simulink model "regenerative_damper_with_battery"  (R2017a)
settings: Solver=ode45  StartTime=0.0  StopTime=0.05  MaxStep=1e-5  RelTol=1e-4
libraries: powerlib_meascontrol x17, fl_lib x12, nesl_utility x11, pe_lib x4, elec_lib x1, powerlib x1
settings Model: Creator=k1506456  LastModifiedBy=k1506456

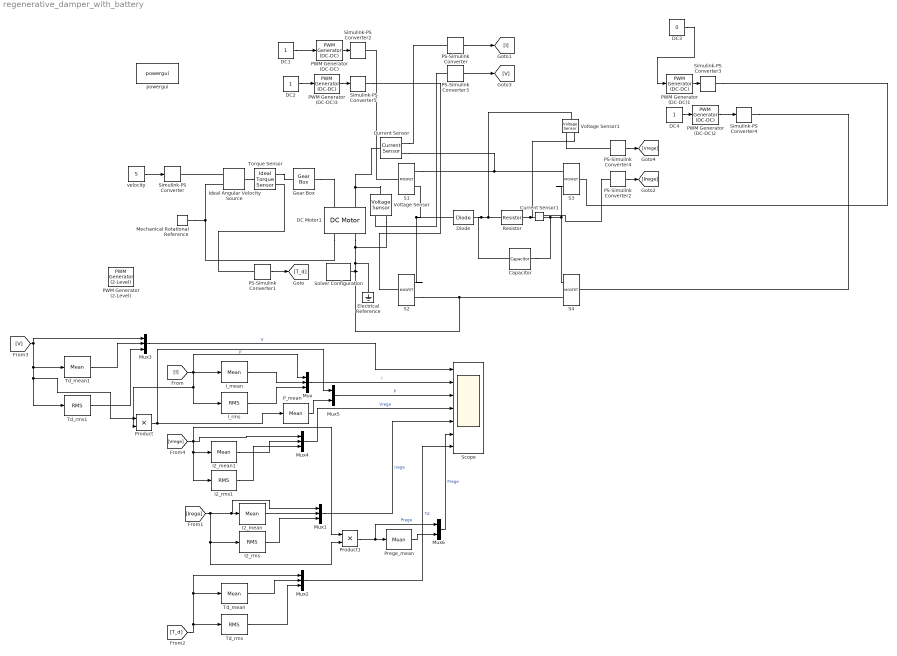
== system regenerative_damper_with_battery ==
  Capacitor : fl_lib/Electrical/Electrical Elements/Capacitor  c=220 uF  r=1e-6 Ohm  g=0 1/Ohm  i_specify=off  i_priority=None  i=0 A  i_nominal_specify=off  i_nominal_unit=A  i_nominal_value=1  v_specify=off  v_priority=None  v=0 V  v_nominal_specify=off  v_nominal_unit=V  v_nominal_value=1  vc_specify=off  vc_priority=High  vc=0 V  vc_nominal_specify=off  vc_nominal_unit=V  vc_nominal_value=1
  Current Sensor : fl_lib/Electrical/Electrical Sensors/Current Sensor
  Current Sensor1 : fl_lib/Electrical/Electrical Sensors/Current Sensor
  DC Motor1 : elec_lib/Actuators & Drivers/Rotational Actuators/DC Motor  parameterization=1  Ra=21.2 Ohm  La=1.37 mH  emf_or_torque=1  Kv=0.00222222 V/rpm  Ki=0.0212 N*m/A  T_stall=2.4e-4 N*m  w_max=1.91e+4 rpm  w_rated=1.5e+4 rpm  P_rated=0.08 W  V_rated=1.5 V  J=4.2 g*cm^2  lam_param=2  lam=0 N*m/(rad/s)  i_noload=8.81 mA  V_i_noload=24 V  speed0=100 rad/s  alpha=0.00393 1/K  Tmeas=25 degC  thermal_mass=100 J/K  initial_temperature=25 degC
  DC1 : Constant
  DC2 : Constant
  DC3 : Constant  Value=0
  DC4 : Constant
  Diode : fl_lib/Electrical/Electrical Elements/Diode  Vf=0.1 V  Ron=0.001 Ohm  Goff=1e-8 1/Ohm  i_specify=off  i_priority=None  i=0 A  i_nominal_specify=off  i_nominal_unit=A  i_nominal_value=1  v_specify=off  v_priority=None  v=0 V  v_nominal_specify=off  v_nominal_unit=V  v_nominal_value=1
  Electrical Reference : fl_lib/Electrical/Electrical Elements/Electrical Reference
  Gear Box : fl_lib/Mechanical/Mechanisms/Gear Box  ratio=1/20  t_in_specify=off  t_in_priority=None  t_in=0 N*m  t_in_nominal_specify=off  t_in_nominal_unit=N*m  t_in_nominal_value=1  t_out_specify=off  t_out_priority=None  t_out=0 N*m  t_out_nominal_specify=off  t_out_nominal_unit=N*m  t_out_nominal_value=1
  I2_mean : powerlib_meascontrol/Measurements/Mean  Freq=100  Vinit=0  Ts=0
  I2_mean1 : powerlib_meascontrol/Measurements/Mean  Freq=50  Vinit=0  Ts=0
  I2_rms : powerlib_meascontrol/Measurements/RMS  TrueRMS=on  Freq=50  RMSInit=0  Ts=0
  I2_rms1 : powerlib_meascontrol/Measurements/RMS  TrueRMS=on  Freq=50  RMSInit=0  Ts=0
  I_mean : powerlib_meascontrol/Measurements/Mean  Freq=50  Vinit=0  Ts=0
  I_rms : powerlib_meascontrol/Measurements/RMS  TrueRMS=on  Freq=50  RMSInit=0  Ts=0
  Ideal Angular Velocity Source : fl_lib/Mechanical/Mechanical Sources/Ideal Angular Velocity Source
  Mechanical Rotational Reference : fl_lib/Mechanical/Rotational Elements/Mechanical Rotational Reference
  Mux{,1..4} (5 alike) : Mux  Inputs=3
  Mux5 : Mux  Inputs=2
  Mux6 : Mux  Inputs=2
  PS-Simulink Converter{,1..4} (5 alike) : nesl_utility/PS-Simulink Converter  PhysicalDomain=network_engine_domain  SubClassName=ps_output  LeftPortType=input  RightPortType=output  PseudoPeriodic=off  Frequencies=[]  Unit=1  AffineConversion=off
  PWM Generator (2-Level) : powerlib_meascontrol/Pulse & Signal Generators/PWM Generator (2-Level)  ModulatorType=Three-phase bridge (6 pulses)  ModulatorMode=Unsynchronized  Fc=5000  Pc=90  nF=27  MinMax="[ -1  1 ]"  SamplingTechnique=Natural  ModulatingSignals=off  m=0.8  Freq=60  Phase=0  Ts=0  ShowCarrierOutport=off
      settings: SourceProductName=Simscape Power Systems
  PWM Generator (DC-DC) : powerlib_meascontrol/Pulse & Signal Generators/PWM Generator (DC-DC)  Fsw=1000  Ts=0
  PWM Generator (DC-DC)1 : powerlib_meascontrol/Pulse & Signal Generators/PWM Generator (DC-DC)  Fsw=1000  Ts=0
  PWM Generator (DC-DC)2 : powerlib_meascontrol/Pulse & Signal Generators/PWM Generator (DC-DC)  Fsw=1000  Ts=0
  PWM Generator (DC-DC)3 : powerlib_meascontrol/Pulse & Signal Generators/PWM Generator (DC-DC)  Fsw=5000  Ts=0
  P_mean : powerlib_meascontrol/Measurements/Mean  Freq=50  Vinit=0  Ts=0
  Prege_mean : powerlib_meascontrol/Measurements/Mean  Freq=50  Vinit=0  Ts=0
  Product : Product
  Product1 : Product
  Resistor : fl_lib/Electrical/Electrical Elements/Resistor  R=21.2 Ohm  i_specify=off  i_priority=None  i=0 A  i_nominal_specify=off  i_nominal_unit=A  i_nominal_value=1  v_specify=off  v_priority=None  v=0 V  v_nominal_specify=off  v_nominal_unit=V  v_nominal_value=1
  S{1..4} (4 alike) : pe_lib/Semiconductors/Fundamental Components/MOSFET  Rds=0.001 Ohm  Goff=1e-6 1/Ohm  Vth=0.8 V  diode_param=2  diode_Vf=0.8 V  diode_Ron=0.001 Ohm  diode_Goff=1e-5 1/Ohm  diode_C=5e-8 F  diode_iRM=-235 A  diode_iF=300 A  diode_idot=-50 A/us  diode_trr_param=1  diode_trr_factor=3  diode_trr=15 us  diode_Qrr=1.5e+3 s*uA  thermal_loss_option=2  Voff=300 V  Tau=1e-4 s  Tj=[ 298.15 398.15 ] K  Iout_scalar=600 A  Eon_scalar=0.02286 J  Eoff_scalar=0.01714 J  Von_scalar=2.7 V  Iout_data=[ 0 10 50 100 200 400 600 ] A  Eon_data=[ 0 2.9e-4 0.00143 0.00286 0.00571 0.01314 0.02286; 0 5.7e-4 0.00263 0.00514 0.01029 0.02057 0.03029 ] J  Eoff_data=[ 0 2.1e-4 0.00107 0.00214 0.00429 0.009859999999999999 0.01714; 0 4.3e-4 0.00197 0.00386 0.00771 0.01543 0.02271 ] J  Von_data=[ 0 1.1 1.3 1.45 1.75 2.25 2.7; 0 1 1.15 1.35 1.7 2.35 3 ] V
      settings: SourceProductName=Simscape Power Systems  SourceProductBaseCode=PS
  Scope : Scope  NumInputPorts=7
  Simulink-PS Converter : nesl_utility/Simulink-PS Converter  PhysicalDomain=network_engine_domain  SubClassName=ps_input  LeftPortType=input  RightPortType=output  PseudoPeriodic=off  Frequencies=[]  NoiseDistribution=none  NoiseParameters=[]  Unit=rad/s  AffineConversion=off  FilteringAndDerivatives=provide  SimscapeFilterOrder=1  InputFilterTimeConstant=0.001  UdotUserProvided=0
  Simulink-PS Converter{2..5} (4 alike) : nesl_utility/Simulink-PS Converter  PhysicalDomain=network_engine_domain  SubClassName=ps_input  LeftPortType=input  RightPortType=output  PseudoPeriodic=off  Frequencies=[]  NoiseDistribution=none  NoiseParameters=[]  Unit=V  AffineConversion=off  FilteringAndDerivatives=provide  SimscapeFilterOrder=1  InputFilterTimeConstant=0.001  UdotUserProvided=0
  Solver Configuration : nesl_utility/Solver Configuration  PhysicalDomain=network_engine_domain  SubClassName=solver  LeftPortType=input  RightPortType=generic  Accelerate=off  Tones=[]  Harmonics=[]  SimulateNoise=off  Profile=off  UseLocalSampling=off  EnableSwitchedLinearOptims=on  FrequencyDomain=off  UseCCode=off  RelTol=0.001  AbsTol=1e-06  MinStep=1e-09  ToWorkspace=off  RevertToSquareIcSolve=off  NumHomotopyIterations=100  PhasorMode=off  PhasorModeNumHarmonics=1  OverrideAbsTol=off  DoDC=off  ResidualTolerance=1e-09  UseLocalSolver=off  LocalSolverChoice=NE_BACKWARD_EULER_ADVANCER  LocalSolverSampleTime=0.001  DoFixedCost=off  MaxNonlinIter=3  MaxModeIter=2  LinearAlgebra=Sparse  DelaysMemoryBudget=1024  AutomaticFiltering=on  FilteringTimeConstant=0.001
  Td_mean : powerlib_meascontrol/Measurements/Mean  Freq=100  Vinit=0  Ts=0
  Td_mean1 : powerlib_meascontrol/Measurements/Mean  Freq=50  Vinit=0  Ts=0
  Td_rms : powerlib_meascontrol/Measurements/RMS  TrueRMS=on  Freq=50  RMSInit=0  Ts=0
  Td_rms1 : powerlib_meascontrol/Measurements/RMS  TrueRMS=on  Freq=50  RMSInit=0  Ts=0
  Torque Sensor : fl_lib/Mechanical/Mechanical Sensors/Ideal Torque Sensor
  Voltage Sensor : fl_lib/Electrical/Electrical Sensors/Voltage Sensor
  Voltage Sensor1 : fl_lib/Electrical/Electrical Sensors/Voltage Sensor
  powergui : powerlib/powergui  Priority=1  SimulationMode=Continuous  SampleTime=5e-6  frequency=60  Iterations=50  frequencyindice=0  Pbase=100e6  ErrMax=1e-4  UnitsV=kV  UnitsW=MW  buscounter=0  FunctionMessages=off  echomessages=off  EnableUseOfTLC=off  CurrentSourceSwitches=off  DisableSnubberDevices=off  DisableRonSwitches=off  DisableVfSwitches=off  DisplayEquations=off  SolverType=Tustin/Backward Euler (TBE)  Interpol=off  ExternalGateDelay=off  methode=off  Ts=100  x0status=blocks  SPID=on  SwTol=0  HookPort=off  RestoreLinks=warning  ResistiveCurrentMeasurement=off  Frange=[0:2:500]  Ylog=off  Xlog=on  ShowGrid=off  save=off  variable=ZData  structure=0  ZoomFFT=off  StartTime=0.0  cycles=1  DisplayStyle=1  fundamental=60  FreqAxis=off  MaxFrequency=1000  frequencyindicesteady=1  RmsSteady=1  display=off
  velocity : Constant  Value=5
  wires:
  velocity/1 -> Simulink-PS Converter/1
  PS-Simulink Converter/1 -> [I]
  PS-Simulink Converter1/1 -> [T_d]
  PWM Generator (DC-DC)/1 -> Simulink-PS Converter2/1
  PWM Generator (DC-DC)1/1 -> Simulink-PS Converter3/1
  PWM Generator (DC-DC)2/1 -> Simulink-PS Converter4/1
  PWM Generator (DC-DC)3/1 -> Simulink-PS Converter5/1
  DC1/1 -> PWM Generator (DC-DC)/1
  DC3/1 -> PWM Generator (DC-DC)1/1
  DC4/1 -> PWM Generator (DC-DC)2/1
  DC2/1 -> PWM Generator (DC-DC)3/1
  PS-Simulink Converter2/1 -> [Irege]
  [I] -> Product/2, I_rms/1, Mux/1, I_mean/1
  [Irege] -> Product1/2, I2_rms/1, Mux1/1, I2_mean/1
  I_mean/1 -> Mux/2
  Mux/1 -> Scope/2  "I"
  [T_d] -> Mux2/1, Td_mean/1, Td_rms/1
  Mux1/1 -> Scope/5  "Irege"
  Mux2/1 -> Scope/7  "Td"
  I2_mean/1 -> Mux1/2
  Td_mean/1 -> Mux2/2
  I2_rms/1 -> Mux1/3
  Td_rms/1 -> Mux2/3
  I_rms/1 -> Mux/3
  PS-Simulink Converter3/1 -> [V]
  [V] -> Mux3/1, Product/1, Td_rms1/1, Td_mean1/1
  Td_mean1/1 -> Mux3/2
  Td_rms1/1 -> Mux3/3
  Mux3/1 -> Scope/1  "V"
  PS-Simulink Converter4/1 -> [Vrege]
  [Vrege] -> Product1/1, Mux4/1, I2_rms1/1, I2_mean1/1
  I2_mean1/1 -> Mux4/2
  I2_rms1/1 -> Mux4/3
  Mux4/1 -> Scope/4  "Vrege"
  Product/1 -> Mux5/1, P_mean/1  "P"
  Product1/1 -> Prege_mean/1, Mux6/1  "Prege"
  P_mean/1 -> Mux5/2
  Mux5/1 -> Scope/3  "P"
  Prege_mean/1 -> Mux6/2
  Mux6/1 -> Scope/6  "Prege"
  connections:
  DC Motor1/RConn2 -- Mechanical Rotational Reference/LConn1 -- Ideal Angular Velocity Source/RConn2
  Ideal Angular Velocity Source/RConn1 -- Simulink-PS Converter/RConn1
  S1/RConn1 -- Current Sensor/RConn2 -- S3/RConn1
  Diode/LConn1 -- S1/RConn2 -- S2/RConn1
  S3/RConn2 -- Capacitor/RConn1 -- Current Sensor1/RConn2 -- S4/RConn1
  S2/RConn2 -- Voltage Sensor/RConn2 -- DC Motor1/RConn1 -- Electrical Reference/LConn1 -- Solver Configuration/RConn1 -- S4/RConn2
  DC Motor1/LConn1 -- Voltage Sensor/LConn1 -- Current Sensor/LConn1
  Current Sensor/RConn1 -- PS-Simulink Converter/LConn1
  PS-Simulink Converter1/LConn1 -- Torque Sensor/RConn2
  S1/LConn1 -- Simulink-PS Converter2/RConn1
  Simulink-PS Converter5/RConn1 -- S2/LConn1
  Simulink-PS Converter4/RConn1 -- S4/LConn1
  Simulink-PS Converter3/RConn1 -- S3/LConn1
  Gear Box/RConn1 -- DC Motor1/LConn2
  PS-Simulink Converter2/LConn1 -- Current Sensor1/RConn1
  PS-Simulink Converter3/LConn1 -- Voltage Sensor/RConn1
  Voltage Sensor1/RConn1 -- PS-Simulink Converter4/LConn1
  Voltage Sensor1/RConn2 -- Current Sensor1/LConn1 -- Resistor/RConn1
  Diode/RConn1 -- Resistor/LConn1 -- Voltage Sensor1/LConn1 -- Capacitor/LConn1
  Ideal Angular Velocity Source/LConn1 -- Torque Sensor/LConn1
  Torque Sensor/RConn1 -- Gear Box/LConn1
